simulink model "test_regler_polbvg_aktoren_sensoren_ansprechen"  (R2016b)
settings: Solver=ode1  StartTime=0.0  StopTime=Inf  FixedStep=0.001  RelTol=1e-3
PostLoadFcn:
  | , if any(exist('dsrtsu_mdlpostloadfcn', 'file') == [2, 3, 6]), try dsrtsu_mdlpostloadfcn('Execute', bdroot); catch fprintf('Error in PostLoadFcn (dsrtsu_mdlpostloadfcn) for model "%s":\n %s\n', bdroot, lasterr); end, end,
undefined symbols (not defined in the file): A_b_angle, A_D, B_b_angle, B_D, C_b_angle, C_D, Continuous, D_b_angle, D_D, matA_g, matA_hub_g, matB, matB_g, matB_hub, matB_hub_g, matC_g, matC_hub_g, matE, matE_hub, matR_ges, matR_hub, reglerhub, system, Time
libraries: rti1202lib_adc_class1 x3, rti1202lib_dac_class1 x2, ctrlSharedLib x2, simulink x1, rtiemclib x1, rti1202lib_base x1
(part 2 of 2)

== system test_regler_polbvg_aktoren_sensoren_ansprechen/RTI Data/RTI Data Store/RTI Data Store ==
  RTI Data Store : Subsystem  mask(RTI_DATA_STORE){}
      mask help:
      | RTI Data Store Block. This block is used by RTI to store internal model dependent data. Deleting this block will result in data loss.
      |
      | NEVER DELETE, COPY, OR MODIFY THIS BLOCK!
      mask Help:
      | RTI Data Store Block. This block is used by RTI to store internal model dependent data. Deleting this block will result in data loss.
      | 
      | NEVER DELETE, COPY, OR MODIFY THIS BLOCK!
      mask Display: text(0.5, 0.5, ' ', 'HorizontalAlignment', 'center');

== system test_regler_polbvg_aktoren_sensoren_ansprechen/RTI Data/RTI Data Store/RTI Data Store/RTI Data Store ==
  RTI Data Store : Subsystem  mask(RTI_DATA_STORE){}
      mask help:
      | RTI Data Store Block. This block is used by RTI to store internal model dependent data. Deleting this block will result in data loss.
      |
      | NEVER DELETE, COPY, OR MODIFY THIS BLOCK!
      mask Help:
      | RTI Data Store Block. This block is used by RTI to store internal model dependent data. Deleting this block will result in data loss.
      | 
      | NEVER DELETE, COPY, OR MODIFY THIS BLOCK!
      mask Display: text(0.5, 0.5, ' ', 'HorizontalAlignment', 'center');

== system test_regler_polbvg_aktoren_sensoren_ansprechen/RTI Data/RTI Data Store/RTI Data Store/RTI Data Store/RTI Data Store ==

== matlab function test_regler_polbvg_aktoren_sensoren_ansprechen/Umrechnung Sensor ==
  data: theta_sensor input; theta output
function theta  = sensorWinkel(theta_sensor)
% berechnet aus dem gemessenen Winkel den tatsächlichen Winkel des
% Lasthebers

% l_verb: Länge des Verbindungsstücks
% l_welle: Abstand der beiden Wellen

% Parameter für die Winkelumrechnung
l_verb = 0.109; % m %
l_welle = 0.0575; % m %

theta = asin(sin(theta_sensor) * (l_verb / sqrt(l_welle^2 + l_verb^2 - (2 * l_verb * l_welle * cos(theta_sensor)))));

== matlab function test_regler_polbvg_aktoren_sensoren_ansprechen/Kalman Filter/Berechnung Systemmatrizen ==
  data: matA_ges output; L input; matB_ges output; matC_ges output; matD_ges output; T_K input; K_K input; R input; ue input; g input
function [matA_ges, matB_ges, matC_ges, matD_ges]  = calcSysMatrixStoerGes(L, T_K, K_K, R, ue, g)

% System ohne Störgrößen
matA = [0 1                           0                   0;
        0 -(T_K^-1)            0                   0;
        0 0                           0                   1;
        0 (T_K*L)^-1    -g*(L^-1)   0];

matB = [0; (2*pi*R*K_K)/(ue*T_K); 0; (-2*pi*R*K_K)/(ue*T_K*L)];

matC = [1 0 0 0; 0 0 1 0];


% Störung: Spannungsoffset
% Einfluss der Störung auf Zustände
matE = matB;

% Störmodell
matA_s = 0; % stückweise konstant
matC_s = 1;

% Modell mit Störung 1
matA_g_1 = [matA                      matE*matC_s;
            zeros(1,size(matA,2))     matA_s];

matB_g_1 = [matB; zeros(1,size(matB,2))];

matC_g_1 = [matC zeros(size(matC,1),1)];


% Störung: Winkeloffset
% Einfluss der Störung auf Zustände
matE = [0; 0; 0; 0; 0]; % kein Einfluss auf Zustände, da Winkeloffset erst am Ausgang wirkt

% Störmodell
matA_s = 0; % stückweise konstant
matC_s = 1;


% Gesamtmodell
matA_ges = [matA_g_1                     matE*matC_s;
            zeros(1,size(matA_g_1,2))    matA_s];

matB_ges = [matB_g_1; zeros(1,size(matB_g_1,2))];

matC_ges = [matC_g_1 [0; 1]]; % nicht wie in bsw. RLM mit Nullen aufgefüllt (s.o.), da Störung erst am Ausgang wirkt

matD_ges = [0; 0];


end
